simulink model "Task07"  (R2022b)
settings: Solver=VariableStepAuto  StartTime=0.0  StopTime=10.0  RelTol=1e-3
libraries: simulink x1
settings Model: Creator=LOQ  LastModifiedBy=LOQ
settings OptimizationCC: ReuseModelBlockBuffer=on
settings RTWCC: GPUComputeCapability=5.0
settings ConfigComp: CovBoundaryAbsTol=1.0e-5

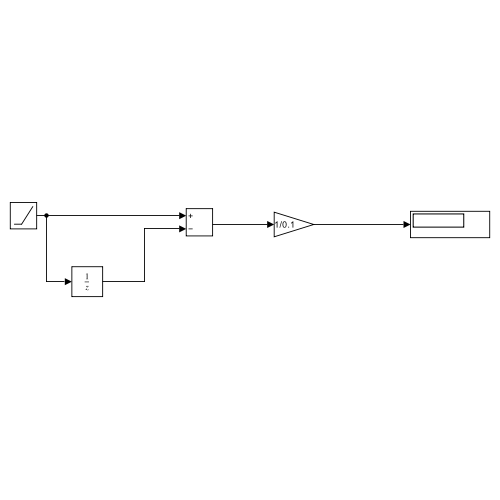
[thumbnail: Simulink's stored preview of the top-level diagram]
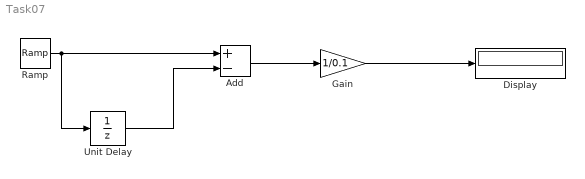
== system Task07 ==
  Add : Sum  Inputs=+-
  Display : Display
  Gain : Gain  Gain=1/0.1
  Ramp : simulink/Sources/Ramp  slope=5  start=0  InitialOutput=0
  Unit Delay : UnitDelay  SampleTime=0.1  HasFrameUpgradeWarning=on
  wires:
  Ramp/1 -> Unit Delay/1, Add/1
  Unit Delay/1 -> Add/2
  Add/1 -> Gain/1
  Gain/1 -> Display/1
